simulink model "RealtimeModel"  (Simulink 7.0)
settings: Solver=FixedStepDiscrete  SolverMode=MultiTasking  StartTime=0.0  StopTime=RunningTime  FixedStep=sample  RelTol=1e-3
values from neighbouring files (symbols this model uses):
  Integrator = InitializeIntegrator(Integrator, Structure)    [RealtimeModel_Setup.m]
  SampleRate = Integrator.Timestep    [RealtimeModel_Setup.m]
  Structure = CalculateMatrices(Structure, Elements)    [RealtimeModel_Setup.m]
undefined symbols (not defined in the file or in its folder): Elements
libraries: simulink x2
(part 4 of 11)

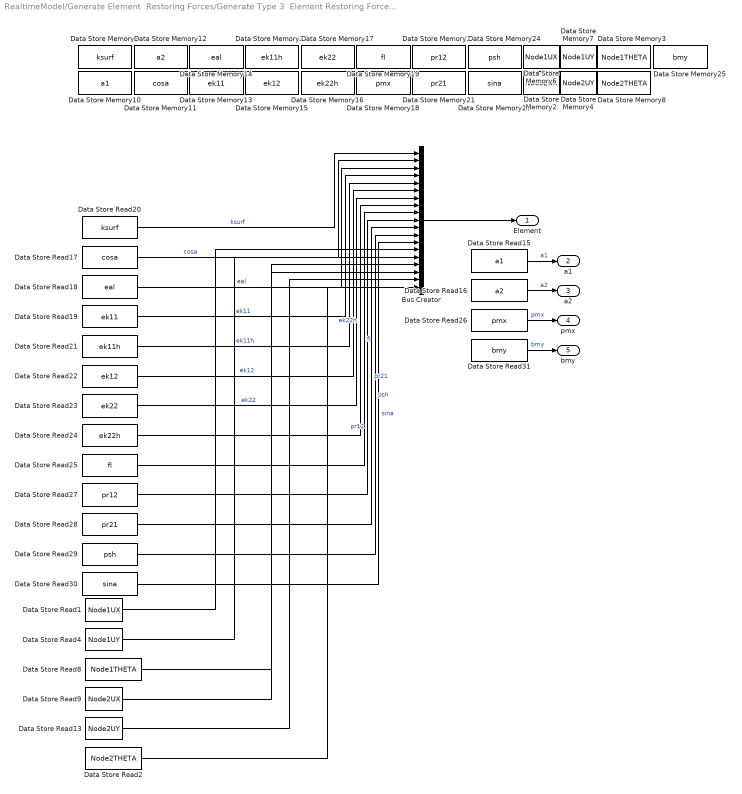
== system RealtimeModel/Generate Element  Restoring Forces/Generate Type 3  Element Restoring Force Element 19/Type 3 Element  ==
  Bus Creator : BusCreator  Inputs=19
  Data Store Memory10 : DataStoreMemory  DataStoreName=a1  InitialValue=Elements{id}.a1  OutDataType=sfix(16)  OutScaling=2^0
  Data Store Memory11 : DataStoreMemory  DataStoreName=cosa  InitialValue=Elements{id}.cosa  OutDataType=sfix(16)  OutScaling=2^0
  Data Store Memory12 : DataStoreMemory  DataStoreName=a2  InitialValue=Elements{id}.a2  OutDataType=sfix(16)  OutScaling=2^0
  Data Store Memory13 : DataStoreMemory  DataStoreName=ek11  InitialValue=Elements{id}.ek11  OutDataType=sfix(16)  OutScaling=2^0
  Data Store Memory14 : DataStoreMemory  DataStoreName=eal  InitialValue=Elements{id}.eal  OutDataType=sfix(16)  OutScaling=2^0
  Data Store Memory15 : DataStoreMemory  DataStoreName=ek12  InitialValue=Elements{id}.ek12  OutDataType=sfix(16)  OutScaling=2^0
  Data Store Memory16 : DataStoreMemory  DataStoreName=ek22h  InitialValue=Elements{id}.ek22h  OutDataType=sfix(16)  OutScaling=2^0
  Data Store Memory17 : DataStoreMemory  DataStoreName=ek22  InitialValue=Elements{id}.ek22  OutDataType=sfix(16)  OutScaling=2^0
  Data Store Memory18 : DataStoreMemory  DataStoreName=pmx  InitialValue=Elements{id}.pmx  OutDataType=sfix(16)  OutScaling=2^0
  Data Store Memory19 : DataStoreMemory  DataStoreName=fl  InitialValue=Elements{id}.fl  OutDataType=sfix(16)  OutScaling=2^0
  Data Store Memory2 : DataStoreMemory  DataStoreName=Node2UX  InitialValue=Elements{id}.Nodes(2).UX  OutDataType=sfix(16)  OutScaling=2^0
  Data Store Memory20 : DataStoreMemory  DataStoreName=ek11h  InitialValue=Elements{id}.ek11h  OutDataType=sfix(16)  OutScaling=2^0
  Data Store Memory21 : DataStoreMemory  DataStoreName=pr21  InitialValue=Elements{id}.pr21  OutDataType=sfix(16)  OutScaling=2^0
  Data Store Memory22 : DataStoreMemory  DataStoreName=pr12  InitialValue=Elements{id}.pr12  OutDataType=sfix(16)  OutScaling=2^0
  Data Store Memory23 : DataStoreMemory  DataStoreName=sina  InitialValue=Elements{id}.sina  OutDataType=sfix(16)  OutScaling=2^0
  Data Store Memory24 : DataStoreMemory  DataStoreName=psh  InitialValue=Elements{id}.psh  OutDataType=sfix(16)  OutScaling=2^0
  Data Store Memory25 : DataStoreMemory  DataStoreName=bmy  InitialValue=Elements{id}.bmy  OutDataType=sfix(16)  OutScaling=2^0
  Data Store Memory3 : DataStoreMemory  DataStoreName=Node1THETA  InitialValue=Elements{id}.Nodes(1).THETA  OutDataType=sfix(16)  OutScaling=2^0
  Data Store Memory4 : DataStoreMemory  DataStoreName=Node2UY  InitialValue=Elements{id}.Nodes(2).UY  OutDataType=sfix(16)  OutScaling=2^0
  Data Store Memory6 : DataStoreMemory  DataStoreName=Node1UX  InitialValue=Elements{id}.Nodes(1).UX  OutDataType=sfix(16)  OutScaling=2^0
  Data Store Memory7 : DataStoreMemory  DataStoreName=Node1UY  InitialValue=Elements{id}.Nodes(1).UY  OutDataType=sfix(16)  OutScaling=2^0
  Data Store Memory8 : DataStoreMemory  DataStoreName=Node2THETA  InitialValue=Elements{id}.Nodes(2).THETA  OutDataType=sfix(16)  OutScaling=2^0
  Data Store Memory9 : DataStoreMemory  DataStoreName=ksurf  InitialValue=Elements{id}.ksurf  OutDataType=sfix(16)  OutScaling=2^0
  Data Store Read1 : DataStoreRead  DataStoreName=Node1UX  SampleTime=-1
  Data Store Read13 : DataStoreRead  DataStoreName=Node2UY  SampleTime=-1
  Data Store Read15 : DataStoreRead  DataStoreName=a1  SampleTime=-1
  Data Store Read16 : DataStoreRead  DataStoreName=a2  SampleTime=-1
  Data Store Read17 : DataStoreRead  DataStoreName=cosa  SampleTime=-1
  Data Store Read18 : DataStoreRead  DataStoreName=eal  SampleTime=-1
  Data Store Read19 : DataStoreRead  DataStoreName=ek11  SampleTime=-1
  Data Store Read2 : DataStoreRead  DataStoreName=Node2THETA  SampleTime=-1
  Data Store Read20 : DataStoreRead  DataStoreName=ksurf  SampleTime=-1
  Data Store Read21 : DataStoreRead  DataStoreName=ek11h  SampleTime=-1
  Data Store Read22 : DataStoreRead  DataStoreName=ek12  SampleTime=-1
  Data Store Read23 : DataStoreRead  DataStoreName=ek22  SampleTime=-1
  Data Store Read24 : DataStoreRead  DataStoreName=ek22h  SampleTime=-1
  Data Store Read25 : DataStoreRead  DataStoreName=fl  SampleTime=-1
  Data Store Read26 : DataStoreRead  DataStoreName=pmx  SampleTime=-1
  Data Store Read27 : DataStoreRead  DataStoreName=pr12  SampleTime=-1
  Data Store Read28 : DataStoreRead  DataStoreName=pr21  SampleTime=-1
  Data Store Read29 : DataStoreRead  DataStoreName=psh  SampleTime=-1
  Data Store Read30 : DataStoreRead  DataStoreName=sina  SampleTime=-1
  Data Store Read31 : DataStoreRead  DataStoreName=bmy  SampleTime=-1
  Data Store Read4 : DataStoreRead  DataStoreName=Node1UY  SampleTime=-1
  Data Store Read8 : DataStoreRead  DataStoreName=Node1THETA  SampleTime=-1
  Data Store Read9 : DataStoreRead  DataStoreName=Node2UX  SampleTime=-1
  Element : Outport  OutDataType=sfix(16)  OutScaling=2^0
  a1 : Outport  Port=2  OutDataType=sfix(16)  OutScaling=2^0
  a2 : Outport  Port=3  OutDataType=sfix(16)  OutScaling=2^0
  pmx : Outport  Port=4  OutDataType=sfix(16)  OutScaling=2^0
  bmy : Outport  Port=5  OutDataType=sfix(16)  OutScaling=2^0
  wires:
  Data Store Read2/1 -> Bus Creator/19
  Data Store Read13/1 -> Bus Creator/18
  Data Store Read9/1 -> Bus Creator/17
  Data Store Read8/1 -> Bus Creator/16
  Data Store Read4/1 -> Bus Creator/15
  Data Store Read1/1 -> Bus Creator/14
  Bus Creator/1 -> Element/1
  Data Store Read20/1 -> Bus Creator/1  "ksurf"
  Data Store Read17/1 -> Bus Creator/2  "cosa"
  Data Store Read18/1 -> Bus Creator/3  "eal"
  Data Store Read19/1 -> Bus Creator/4  "ek11"
  Data Store Read21/1 -> Bus Creator/5  "ek11h"
  Data Store Read22/1 -> Bus Creator/6  "ek12"
  Data Store Read23/1 -> Bus Creator/7  "ek22"
  Data Store Read24/1 -> Bus Creator/8  "ek22h"
  Data Store Read25/1 -> Bus Creator/9  "fl"
  Data Store Read27/1 -> Bus Creator/10  "pr12"
  Data Store Read28/1 -> Bus Creator/11  "pr21"
  Data Store Read29/1 -> Bus Creator/12  "psh"
  Data Store Read30/1 -> Bus Creator/13  "sina"
  Data Store Read15/1 -> a1/1  "a1"
  Data Store Read16/1 -> a2/1  "a2"
  Data Store Read26/1 -> pmx/1  "pmx"
  Data Store Read31/1 -> bmy/1  "bmy"

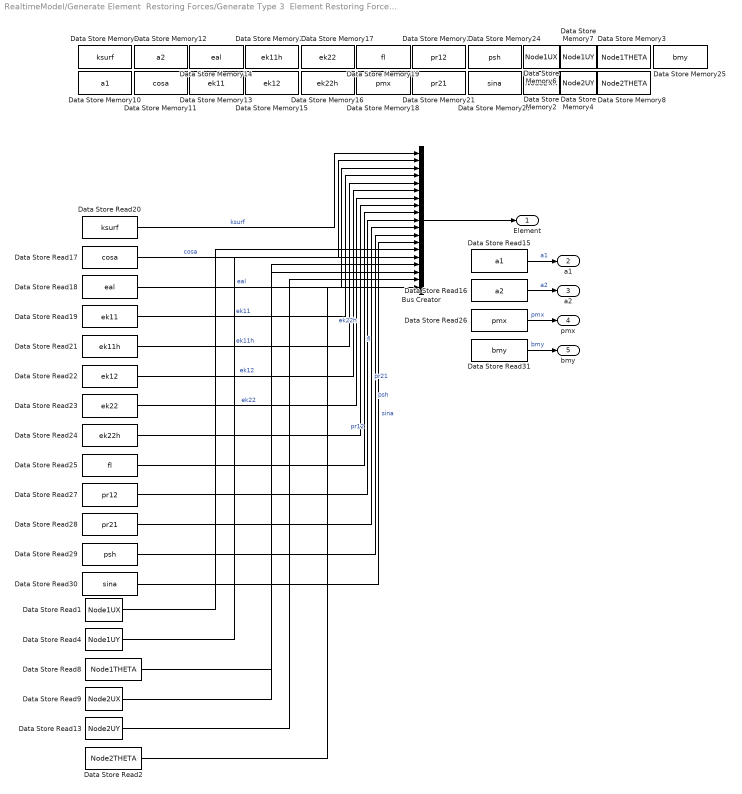
== system RealtimeModel/Generate Element  Restoring Forces/Generate Type 3  Element Restoring Force Element 2/Type 3 Element  ==
  Bus Creator : BusCreator  Inputs=19
  Data Store Memory10 : DataStoreMemory  DataStoreName=a1  InitialValue=Elements{id}.a1  OutDataType=sfix(16)  OutScaling=2^0
  Data Store Memory11 : DataStoreMemory  DataStoreName=cosa  InitialValue=Elements{id}.cosa  OutDataType=sfix(16)  OutScaling=2^0
  Data Store Memory12 : DataStoreMemory  DataStoreName=a2  InitialValue=Elements{id}.a2  OutDataType=sfix(16)  OutScaling=2^0
  Data Store Memory13 : DataStoreMemory  DataStoreName=ek11  InitialValue=Elements{id}.ek11  OutDataType=sfix(16)  OutScaling=2^0
  Data Store Memory14 : DataStoreMemory  DataStoreName=eal  InitialValue=Elements{id}.eal  OutDataType=sfix(16)  OutScaling=2^0
  Data Store Memory15 : DataStoreMemory  DataStoreName=ek12  InitialValue=Elements{id}.ek12  OutDataType=sfix(16)  OutScaling=2^0
  Data Store Memory16 : DataStoreMemory  DataStoreName=ek22h  InitialValue=Elements{id}.ek22h  OutDataType=sfix(16)  OutScaling=2^0
  Data Store Memory17 : DataStoreMemory  DataStoreName=ek22  InitialValue=Elements{id}.ek22  OutDataType=sfix(16)  OutScaling=2^0
  Data Store Memory18 : DataStoreMemory  DataStoreName=pmx  InitialValue=Elements{id}.pmx  OutDataType=sfix(16)  OutScaling=2^0
  Data Store Memory19 : DataStoreMemory  DataStoreName=fl  InitialValue=Elements{id}.fl  OutDataType=sfix(16)  OutScaling=2^0
  Data Store Memory2 : DataStoreMemory  DataStoreName=Node2UX  InitialValue=Elements{id}.Nodes(2).UX  OutDataType=sfix(16)  OutScaling=2^0
  Data Store Memory20 : DataStoreMemory  DataStoreName=ek11h  InitialValue=Elements{id}.ek11h  OutDataType=sfix(16)  OutScaling=2^0
  Data Store Memory21 : DataStoreMemory  DataStoreName=pr21  InitialValue=Elements{id}.pr21  OutDataType=sfix(16)  OutScaling=2^0
  Data Store Memory22 : DataStoreMemory  DataStoreName=pr12  InitialValue=Elements{id}.pr12  OutDataType=sfix(16)  OutScaling=2^0
  Data Store Memory23 : DataStoreMemory  DataStoreName=sina  InitialValue=Elements{id}.sina  OutDataType=sfix(16)  OutScaling=2^0
  Data Store Memory24 : DataStoreMemory  DataStoreName=psh  InitialValue=Elements{id}.psh  OutDataType=sfix(16)  OutScaling=2^0
  Data Store Memory25 : DataStoreMemory  DataStoreName=bmy  InitialValue=Elements{id}.bmy  OutDataType=sfix(16)  OutScaling=2^0
  Data Store Memory3 : DataStoreMemory  DataStoreName=Node1THETA  InitialValue=Elements{id}.Nodes(1).THETA  OutDataType=sfix(16)  OutScaling=2^0
  Data Store Memory4 : DataStoreMemory  DataStoreName=Node2UY  InitialValue=Elements{id}.Nodes(2).UY  OutDataType=sfix(16)  OutScaling=2^0
  Data Store Memory6 : DataStoreMemory  DataStoreName=Node1UX  InitialValue=Elements{id}.Nodes(1).UX  OutDataType=sfix(16)  OutScaling=2^0
  Data Store Memory7 : DataStoreMemory  DataStoreName=Node1UY  InitialValue=Elements{id}.Nodes(1).UY  OutDataType=sfix(16)  OutScaling=2^0
  Data Store Memory8 : DataStoreMemory  DataStoreName=Node2THETA  InitialValue=Elements{id}.Nodes(2).THETA  OutDataType=sfix(16)  OutScaling=2^0
  Data Store Memory9 : DataStoreMemory  DataStoreName=ksurf  InitialValue=Elements{id}.ksurf  OutDataType=sfix(16)  OutScaling=2^0
  Data Store Read1 : DataStoreRead  DataStoreName=Node1UX  SampleTime=-1
  Data Store Read13 : DataStoreRead  DataStoreName=Node2UY  SampleTime=-1
  Data Store Read15 : DataStoreRead  DataStoreName=a1  SampleTime=-1
  Data Store Read16 : DataStoreRead  DataStoreName=a2  SampleTime=-1
  Data Store Read17 : DataStoreRead  DataStoreName=cosa  SampleTime=-1
  Data Store Read18 : DataStoreRead  DataStoreName=eal  SampleTime=-1
  Data Store Read19 : DataStoreRead  DataStoreName=ek11  SampleTime=-1
  Data Store Read2 : DataStoreRead  DataStoreName=Node2THETA  SampleTime=-1
  Data Store Read20 : DataStoreRead  DataStoreName=ksurf  SampleTime=-1
  Data Store Read21 : DataStoreRead  DataStoreName=ek11h  SampleTime=-1
  Data Store Read22 : DataStoreRead  DataStoreName=ek12  SampleTime=-1
  Data Store Read23 : DataStoreRead  DataStoreName=ek22  SampleTime=-1
  Data Store Read24 : DataStoreRead  DataStoreName=ek22h  SampleTime=-1
  Data Store Read25 : DataStoreRead  DataStoreName=fl  SampleTime=-1
  Data Store Read26 : DataStoreRead  DataStoreName=pmx  SampleTime=-1
  Data Store Read27 : DataStoreRead  DataStoreName=pr12  SampleTime=-1
  Data Store Read28 : DataStoreRead  DataStoreName=pr21  SampleTime=-1
  Data Store Read29 : DataStoreRead  DataStoreName=psh  SampleTime=-1
  Data Store Read30 : DataStoreRead  DataStoreName=sina  SampleTime=-1
  Data Store Read31 : DataStoreRead  DataStoreName=bmy  SampleTime=-1
  Data Store Read4 : DataStoreRead  DataStoreName=Node1UY  SampleTime=-1
  Data Store Read8 : DataStoreRead  DataStoreName=Node1THETA  SampleTime=-1
  Data Store Read9 : DataStoreRead  DataStoreName=Node2UX  SampleTime=-1
  Element : Outport  OutDataType=sfix(16)  OutScaling=2^0
  a1 : Outport  Port=2  OutDataType=sfix(16)  OutScaling=2^0
  a2 : Outport  Port=3  OutDataType=sfix(16)  OutScaling=2^0
  pmx : Outport  Port=4  OutDataType=sfix(16)  OutScaling=2^0
  bmy : Outport  Port=5  OutDataType=sfix(16)  OutScaling=2^0
  wires:
  Data Store Read31/1 -> bmy/1  "bmy"
  Data Store Read26/1 -> pmx/1  "pmx"
  Data Store Read16/1 -> a2/1  "a2"
  Data Store Read15/1 -> a1/1  "a1"
  Data Store Read30/1 -> Bus Creator/13  "sina"
  Data Store Read29/1 -> Bus Creator/12  "psh"
  Data Store Read28/1 -> Bus Creator/11  "pr21"
  Data Store Read27/1 -> Bus Creator/10  "pr12"
  Data Store Read25/1 -> Bus Creator/9  "fl"
  Data Store Read24/1 -> Bus Creator/8  "ek22h"
  Data Store Read23/1 -> Bus Creator/7  "ek22"
  Data Store Read22/1 -> Bus Creator/6  "ek12"
  Data Store Read21/1 -> Bus Creator/5  "ek11h"
  Data Store Read19/1 -> Bus Creator/4  "ek11"
  Data Store Read18/1 -> Bus Creator/3  "eal"
  Data Store Read17/1 -> Bus Creator/2  "cosa"
  Data Store Read20/1 -> Bus Creator/1  "ksurf"
  Bus Creator/1 -> Element/1
  Data Store Read1/1 -> Bus Creator/14
  Data Store Read4/1 -> Bus Creator/15
  Data Store Read8/1 -> Bus Creator/16
  Data Store Read9/1 -> Bus Creator/17
  Data Store Read13/1 -> Bus Creator/18
  Data Store Read2/1 -> Bus Creator/19

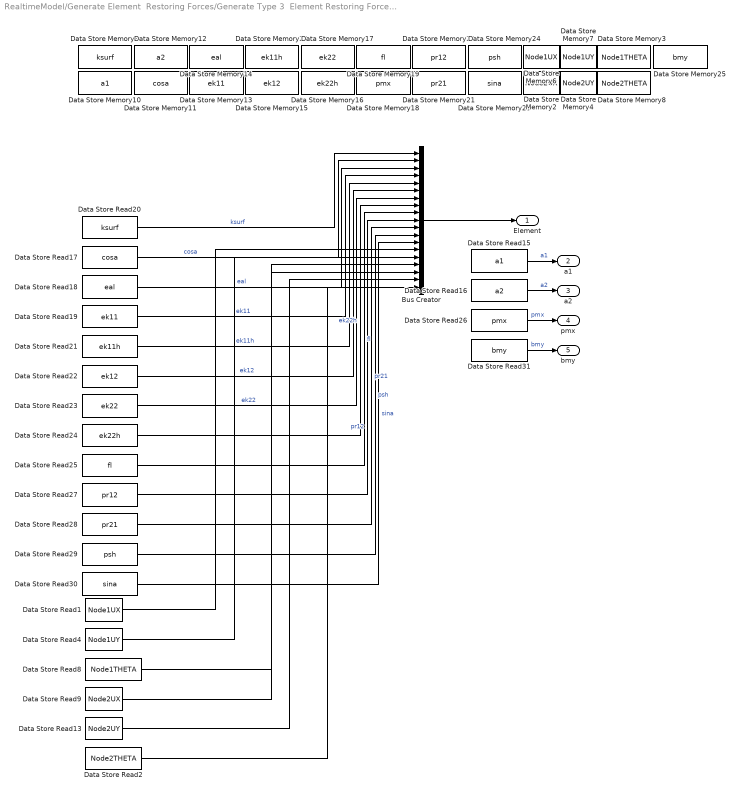
== system RealtimeModel/Generate Element  Restoring Forces/Generate Type 3  Element Restoring Force Element 21/Type 3 Element  ==
  Bus Creator : BusCreator  Inputs=19
  Data Store Memory10 : DataStoreMemory  DataStoreName=a1  InitialValue=Elements{id}.a1  OutDataType=sfix(16)  OutScaling=2^0
  Data Store Memory11 : DataStoreMemory  DataStoreName=cosa  InitialValue=Elements{id}.cosa  OutDataType=sfix(16)  OutScaling=2^0
  Data Store Memory12 : DataStoreMemory  DataStoreName=a2  InitialValue=Elements{id}.a2  OutDataType=sfix(16)  OutScaling=2^0
  Data Store Memory13 : DataStoreMemory  DataStoreName=ek11  InitialValue=Elements{id}.ek11  OutDataType=sfix(16)  OutScaling=2^0
  Data Store Memory14 : DataStoreMemory  DataStoreName=eal  InitialValue=Elements{id}.eal  OutDataType=sfix(16)  OutScaling=2^0
  Data Store Memory15 : DataStoreMemory  DataStoreName=ek12  InitialValue=Elements{id}.ek12  OutDataType=sfix(16)  OutScaling=2^0
  Data Store Memory16 : DataStoreMemory  DataStoreName=ek22h  InitialValue=Elements{id}.ek22h  OutDataType=sfix(16)  OutScaling=2^0
  Data Store Memory17 : DataStoreMemory  DataStoreName=ek22  InitialValue=Elements{id}.ek22  OutDataType=sfix(16)  OutScaling=2^0
  Data Store Memory18 : DataStoreMemory  DataStoreName=pmx  InitialValue=Elements{id}.pmx  OutDataType=sfix(16)  OutScaling=2^0
  Data Store Memory19 : DataStoreMemory  DataStoreName=fl  InitialValue=Elements{id}.fl  OutDataType=sfix(16)  OutScaling=2^0
  Data Store Memory2 : DataStoreMemory  DataStoreName=Node2UX  InitialValue=Elements{id}.Nodes(2).UX  OutDataType=sfix(16)  OutScaling=2^0
  Data Store Memory20 : DataStoreMemory  DataStoreName=ek11h  InitialValue=Elements{id}.ek11h  OutDataType=sfix(16)  OutScaling=2^0
  Data Store Memory21 : DataStoreMemory  DataStoreName=pr21  InitialValue=Elements{id}.pr21  OutDataType=sfix(16)  OutScaling=2^0
  Data Store Memory22 : DataStoreMemory  DataStoreName=pr12  InitialValue=Elements{id}.pr12  OutDataType=sfix(16)  OutScaling=2^0
  Data Store Memory23 : DataStoreMemory  DataStoreName=sina  InitialValue=Elements{id}.sina  OutDataType=sfix(16)  OutScaling=2^0
  Data Store Memory24 : DataStoreMemory  DataStoreName=psh  InitialValue=Elements{id}.psh  OutDataType=sfix(16)  OutScaling=2^0
  Data Store Memory25 : DataStoreMemory  DataStoreName=bmy  InitialValue=Elements{id}.bmy  OutDataType=sfix(16)  OutScaling=2^0
  Data Store Memory3 : DataStoreMemory  DataStoreName=Node1THETA  InitialValue=Elements{id}.Nodes(1).THETA  OutDataType=sfix(16)  OutScaling=2^0
  Data Store Memory4 : DataStoreMemory  DataStoreName=Node2UY  InitialValue=Elements{id}.Nodes(2).UY  OutDataType=sfix(16)  OutScaling=2^0
  Data Store Memory6 : DataStoreMemory  DataStoreName=Node1UX  InitialValue=Elements{id}.Nodes(1).UX  OutDataType=sfix(16)  OutScaling=2^0
  Data Store Memory7 : DataStoreMemory  DataStoreName=Node1UY  InitialValue=Elements{id}.Nodes(1).UY  OutDataType=sfix(16)  OutScaling=2^0
  Data Store Memory8 : DataStoreMemory  DataStoreName=Node2THETA  InitialValue=Elements{id}.Nodes(2).THETA  OutDataType=sfix(16)  OutScaling=2^0
  Data Store Memory9 : DataStoreMemory  DataStoreName=ksurf  InitialValue=Elements{id}.ksurf  OutDataType=sfix(16)  OutScaling=2^0
  Data Store Read1 : DataStoreRead  DataStoreName=Node1UX  SampleTime=-1
  Data Store Read13 : DataStoreRead  DataStoreName=Node2UY  SampleTime=-1
  Data Store Read15 : DataStoreRead  DataStoreName=a1  SampleTime=-1
  Data Store Read16 : DataStoreRead  DataStoreName=a2  SampleTime=-1
  Data Store Read17 : DataStoreRead  DataStoreName=cosa  SampleTime=-1
  Data Store Read18 : DataStoreRead  DataStoreName=eal  SampleTime=-1
  Data Store Read19 : DataStoreRead  DataStoreName=ek11  SampleTime=-1
  Data Store Read2 : DataStoreRead  DataStoreName=Node2THETA  SampleTime=-1
  Data Store Read20 : DataStoreRead  DataStoreName=ksurf  SampleTime=-1
  Data Store Read21 : DataStoreRead  DataStoreName=ek11h  SampleTime=-1
  Data Store Read22 : DataStoreRead  DataStoreName=ek12  SampleTime=-1
  Data Store Read23 : DataStoreRead  DataStoreName=ek22  SampleTime=-1
  Data Store Read24 : DataStoreRead  DataStoreName=ek22h  SampleTime=-1
  Data Store Read25 : DataStoreRead  DataStoreName=fl  SampleTime=-1
  Data Store Read26 : DataStoreRead  DataStoreName=pmx  SampleTime=-1
  Data Store Read27 : DataStoreRead  DataStoreName=pr12  SampleTime=-1
  Data Store Read28 : DataStoreRead  DataStoreName=pr21  SampleTime=-1
  Data Store Read29 : DataStoreRead  DataStoreName=psh  SampleTime=-1
  Data Store Read30 : DataStoreRead  DataStoreName=sina  SampleTime=-1
  Data Store Read31 : DataStoreRead  DataStoreName=bmy  SampleTime=-1
  Data Store Read4 : DataStoreRead  DataStoreName=Node1UY  SampleTime=-1
  Data Store Read8 : DataStoreRead  DataStoreName=Node1THETA  SampleTime=-1
  Data Store Read9 : DataStoreRead  DataStoreName=Node2UX  SampleTime=-1
  Element : Outport  OutDataType=sfix(16)  OutScaling=2^0
  a1 : Outport  Port=2  OutDataType=sfix(16)  OutScaling=2^0
  a2 : Outport  Port=3  OutDataType=sfix(16)  OutScaling=2^0
  pmx : Outport  Port=4  OutDataType=sfix(16)  OutScaling=2^0
  bmy : Outport  Port=5  OutDataType=sfix(16)  OutScaling=2^0
  wires:
  Data Store Read2/1 -> Bus Creator/19
  Data Store Read13/1 -> Bus Creator/18
  Data Store Read9/1 -> Bus Creator/17
  Data Store Read8/1 -> Bus Creator/16
  Data Store Read4/1 -> Bus Creator/15
  Data Store Read1/1 -> Bus Creator/14
  Bus Creator/1 -> Element/1
  Data Store Read20/1 -> Bus Creator/1  "ksurf"
  Data Store Read17/1 -> Bus Creator/2  "cosa"
  Data Store Read18/1 -> Bus Creator/3  "eal"
  Data Store Read19/1 -> Bus Creator/4  "ek11"
  Data Store Read21/1 -> Bus Creator/5  "ek11h"
  Data Store Read22/1 -> Bus Creator/6  "ek12"
  Data Store Read23/1 -> Bus Creator/7  "ek22"
  Data Store Read24/1 -> Bus Creator/8  "ek22h"
  Data Store Read25/1 -> Bus Creator/9  "fl"
  Data Store Read27/1 -> Bus Creator/10  "pr12"
  Data Store Read28/1 -> Bus Creator/11  "pr21"
  Data Store Read29/1 -> Bus Creator/12  "psh"
  Data Store Read30/1 -> Bus Creator/13  "sina"
  Data Store Read15/1 -> a1/1  "a1"
  Data Store Read16/1 -> a2/1  "a2"
  Data Store Read26/1 -> pmx/1  "pmx"
  Data Store Read31/1 -> bmy/1  "bmy"

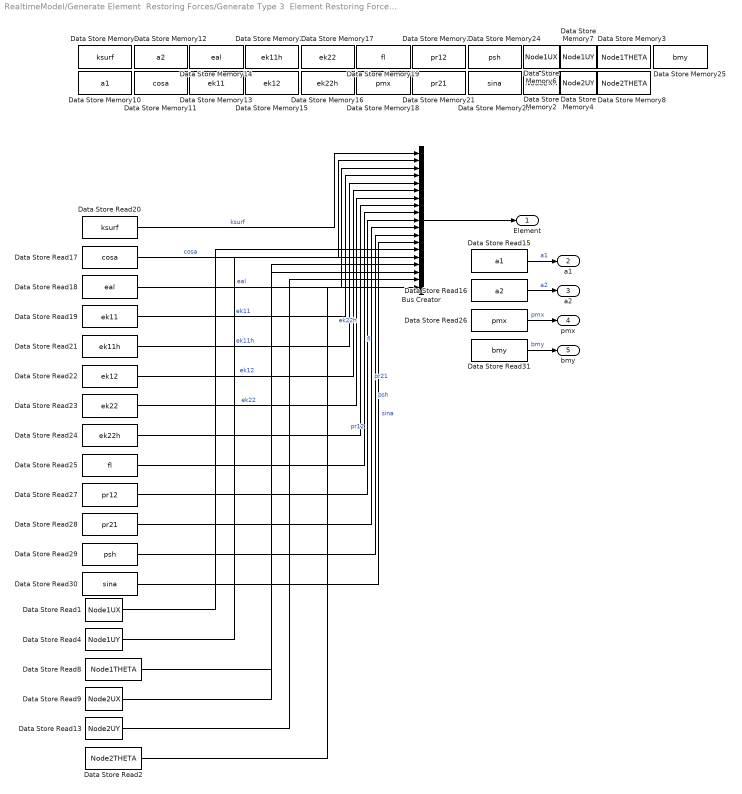
== system RealtimeModel/Generate Element  Restoring Forces/Generate Type 3  Element Restoring Force Element 22/Type 3 Element  ==
  Bus Creator : BusCreator  Inputs=19
  Data Store Memory10 : DataStoreMemory  DataStoreName=a1  InitialValue=Elements{id}.a1  OutDataType=sfix(16)  OutScaling=2^0
  Data Store Memory11 : DataStoreMemory  DataStoreName=cosa  InitialValue=Elements{id}.cosa  OutDataType=sfix(16)  OutScaling=2^0
  Data Store Memory12 : DataStoreMemory  DataStoreName=a2  InitialValue=Elements{id}.a2  OutDataType=sfix(16)  OutScaling=2^0
  Data Store Memory13 : DataStoreMemory  DataStoreName=ek11  InitialValue=Elements{id}.ek11  OutDataType=sfix(16)  OutScaling=2^0
  Data Store Memory14 : DataStoreMemory  DataStoreName=eal  InitialValue=Elements{id}.eal  OutDataType=sfix(16)  OutScaling=2^0
  Data Store Memory15 : DataStoreMemory  DataStoreName=ek12  InitialValue=Elements{id}.ek12  OutDataType=sfix(16)  OutScaling=2^0
  Data Store Memory16 : DataStoreMemory  DataStoreName=ek22h  InitialValue=Elements{id}.ek22h  OutDataType=sfix(16)  OutScaling=2^0
  Data Store Memory17 : DataStoreMemory  DataStoreName=ek22  InitialValue=Elements{id}.ek22  OutDataType=sfix(16)  OutScaling=2^0
  Data Store Memory18 : DataStoreMemory  DataStoreName=pmx  InitialValue=Elements{id}.pmx  OutDataType=sfix(16)  OutScaling=2^0
  Data Store Memory19 : DataStoreMemory  DataStoreName=fl  InitialValue=Elements{id}.fl  OutDataType=sfix(16)  OutScaling=2^0
  Data Store Memory2 : DataStoreMemory  DataStoreName=Node2UX  InitialValue=Elements{id}.Nodes(2).UX  OutDataType=sfix(16)  OutScaling=2^0
  Data Store Memory20 : DataStoreMemory  DataStoreName=ek11h  InitialValue=Elements{id}.ek11h  OutDataType=sfix(16)  OutScaling=2^0
  Data Store Memory21 : DataStoreMemory  DataStoreName=pr21  InitialValue=Elements{id}.pr21  OutDataType=sfix(16)  OutScaling=2^0
  Data Store Memory22 : DataStoreMemory  DataStoreName=pr12  InitialValue=Elements{id}.pr12  OutDataType=sfix(16)  OutScaling=2^0
  Data Store Memory23 : DataStoreMemory  DataStoreName=sina  InitialValue=Elements{id}.sina  OutDataType=sfix(16)  OutScaling=2^0
  Data Store Memory24 : DataStoreMemory  DataStoreName=psh  InitialValue=Elements{id}.psh  OutDataType=sfix(16)  OutScaling=2^0
  Data Store Memory25 : DataStoreMemory  DataStoreName=bmy  InitialValue=Elements{id}.bmy  OutDataType=sfix(16)  OutScaling=2^0
  Data Store Memory3 : DataStoreMemory  DataStoreName=Node1THETA  InitialValue=Elements{id}.Nodes(1).THETA  OutDataType=sfix(16)  OutScaling=2^0
  Data Store Memory4 : DataStoreMemory  DataStoreName=Node2UY  InitialValue=Elements{id}.Nodes(2).UY  OutDataType=sfix(16)  OutScaling=2^0
  Data Store Memory6 : DataStoreMemory  DataStoreName=Node1UX  InitialValue=Elements{id}.Nodes(1).UX  OutDataType=sfix(16)  OutScaling=2^0
  Data Store Memory7 : DataStoreMemory  DataStoreName=Node1UY  InitialValue=Elements{id}.Nodes(1).UY  OutDataType=sfix(16)  OutScaling=2^0
  Data Store Memory8 : DataStoreMemory  DataStoreName=Node2THETA  InitialValue=Elements{id}.Nodes(2).THETA  OutDataType=sfix(16)  OutScaling=2^0
  Data Store Memory9 : DataStoreMemory  DataStoreName=ksurf  InitialValue=Elements{id}.ksurf  OutDataType=sfix(16)  OutScaling=2^0
  Data Store Read1 : DataStoreRead  DataStoreName=Node1UX  SampleTime=-1
  Data Store Read13 : DataStoreRead  DataStoreName=Node2UY  SampleTime=-1
  Data Store Read15 : DataStoreRead  DataStoreName=a1  SampleTime=-1
  Data Store Read16 : DataStoreRead  DataStoreName=a2  SampleTime=-1
  Data Store Read17 : DataStoreRead  DataStoreName=cosa  SampleTime=-1
  Data Store Read18 : DataStoreRead  DataStoreName=eal  SampleTime=-1
  Data Store Read19 : DataStoreRead  DataStoreName=ek11  SampleTime=-1
  Data Store Read2 : DataStoreRead  DataStoreName=Node2THETA  SampleTime=-1
  Data Store Read20 : DataStoreRead  DataStoreName=ksurf  SampleTime=-1
  Data Store Read21 : DataStoreRead  DataStoreName=ek11h  SampleTime=-1
  Data Store Read22 : DataStoreRead  DataStoreName=ek12  SampleTime=-1
  Data Store Read23 : DataStoreRead  DataStoreName=ek22  SampleTime=-1
  Data Store Read24 : DataStoreRead  DataStoreName=ek22h  SampleTime=-1
  Data Store Read25 : DataStoreRead  DataStoreName=fl  SampleTime=-1
  Data Store Read26 : DataStoreRead  DataStoreName=pmx  SampleTime=-1
  Data Store Read27 : DataStoreRead  DataStoreName=pr12  SampleTime=-1
  Data Store Read28 : DataStoreRead  DataStoreName=pr21  SampleTime=-1
  Data Store Read29 : DataStoreRead  DataStoreName=psh  SampleTime=-1
  Data Store Read30 : DataStoreRead  DataStoreName=sina  SampleTime=-1
  Data Store Read31 : DataStoreRead  DataStoreName=bmy  SampleTime=-1
  Data Store Read4 : DataStoreRead  DataStoreName=Node1UY  SampleTime=-1
  Data Store Read8 : DataStoreRead  DataStoreName=Node1THETA  SampleTime=-1
  Data Store Read9 : DataStoreRead  DataStoreName=Node2UX  SampleTime=-1
  Element : Outport  OutDataType=sfix(16)  OutScaling=2^0
  a1 : Outport  Port=2  OutDataType=sfix(16)  OutScaling=2^0
  a2 : Outport  Port=3  OutDataType=sfix(16)  OutScaling=2^0
  pmx : Outport  Port=4  OutDataType=sfix(16)  OutScaling=2^0
  bmy : Outport  Port=5  OutDataType=sfix(16)  OutScaling=2^0
  wires:
  Data Store Read31/1 -> bmy/1  "bmy"
  Data Store Read26/1 -> pmx/1  "pmx"
  Data Store Read16/1 -> a2/1  "a2"
  Data Store Read15/1 -> a1/1  "a1"
  Data Store Read30/1 -> Bus Creator/13  "sina"
  Data Store Read29/1 -> Bus Creator/12  "psh"
  Data Store Read28/1 -> Bus Creator/11  "pr21"
  Data Store Read27/1 -> Bus Creator/10  "pr12"
  Data Store Read25/1 -> Bus Creator/9  "fl"
  Data Store Read24/1 -> Bus Creator/8  "ek22h"
  Data Store Read23/1 -> Bus Creator/7  "ek22"
  Data Store Read22/1 -> Bus Creator/6  "ek12"
  Data Store Read21/1 -> Bus Creator/5  "ek11h"
  Data Store Read19/1 -> Bus Creator/4  "ek11"
  Data Store Read18/1 -> Bus Creator/3  "eal"
  Data Store Read17/1 -> Bus Creator/2  "cosa"
  Data Store Read20/1 -> Bus Creator/1  "ksurf"
  Bus Creator/1 -> Element/1
  Data Store Read1/1 -> Bus Creator/14
  Data Store Read4/1 -> Bus Creator/15
  Data Store Read8/1 -> Bus Creator/16
  Data Store Read9/1 -> Bus Creator/17
  Data Store Read13/1 -> Bus Creator/18
  Data Store Read2/1 -> Bus Creator/19

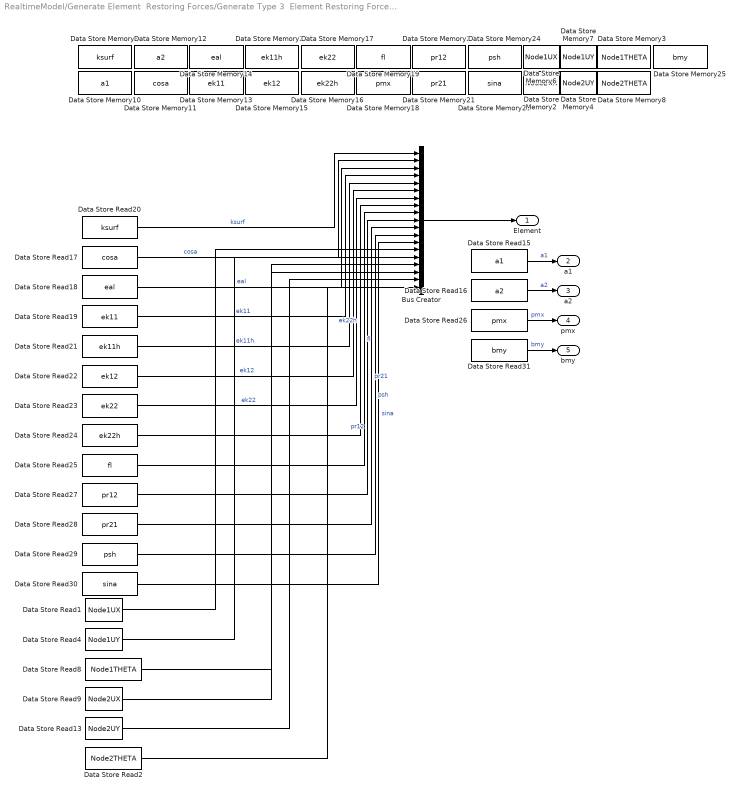
== system RealtimeModel/Generate Element  Restoring Forces/Generate Type 3  Element Restoring Force Element 24/Type 3 Element  ==
  Bus Creator : BusCreator  Inputs=19
  Data Store Memory10 : DataStoreMemory  DataStoreName=a1  InitialValue=Elements{id}.a1  OutDataType=sfix(16)  OutScaling=2^0
  Data Store Memory11 : DataStoreMemory  DataStoreName=cosa  InitialValue=Elements{id}.cosa  OutDataType=sfix(16)  OutScaling=2^0
  Data Store Memory12 : DataStoreMemory  DataStoreName=a2  InitialValue=Elements{id}.a2  OutDataType=sfix(16)  OutScaling=2^0
  Data Store Memory13 : DataStoreMemory  DataStoreName=ek11  InitialValue=Elements{id}.ek11  OutDataType=sfix(16)  OutScaling=2^0
  Data Store Memory14 : DataStoreMemory  DataStoreName=eal  InitialValue=Elements{id}.eal  OutDataType=sfix(16)  OutScaling=2^0
  Data Store Memory15 : DataStoreMemory  DataStoreName=ek12  InitialValue=Elements{id}.ek12  OutDataType=sfix(16)  OutScaling=2^0
  Data Store Memory16 : DataStoreMemory  DataStoreName=ek22h  InitialValue=Elements{id}.ek22h  OutDataType=sfix(16)  OutScaling=2^0
  Data Store Memory17 : DataStoreMemory  DataStoreName=ek22  InitialValue=Elements{id}.ek22  OutDataType=sfix(16)  OutScaling=2^0
  Data Store Memory18 : DataStoreMemory  DataStoreName=pmx  InitialValue=Elements{id}.pmx  OutDataType=sfix(16)  OutScaling=2^0
  Data Store Memory19 : DataStoreMemory  DataStoreName=fl  InitialValue=Elements{id}.fl  OutDataType=sfix(16)  OutScaling=2^0
  Data Store Memory2 : DataStoreMemory  DataStoreName=Node2UX  InitialValue=Elements{id}.Nodes(2).UX  OutDataType=sfix(16)  OutScaling=2^0
  Data Store Memory20 : DataStoreMemory  DataStoreName=ek11h  InitialValue=Elements{id}.ek11h  OutDataType=sfix(16)  OutScaling=2^0
  Data Store Memory21 : DataStoreMemory  DataStoreName=pr21  InitialValue=Elements{id}.pr21  OutDataType=sfix(16)  OutScaling=2^0
  Data Store Memory22 : DataStoreMemory  DataStoreName=pr12  InitialValue=Elements{id}.pr12  OutDataType=sfix(16)  OutScaling=2^0
  Data Store Memory23 : DataStoreMemory  DataStoreName=sina  InitialValue=Elements{id}.sina  OutDataType=sfix(16)  OutScaling=2^0
  Data Store Memory24 : DataStoreMemory  DataStoreName=psh  InitialValue=Elements{id}.psh  OutDataType=sfix(16)  OutScaling=2^0
  Data Store Memory25 : DataStoreMemory  DataStoreName=bmy  InitialValue=Elements{id}.bmy  OutDataType=sfix(16)  OutScaling=2^0
  Data Store Memory3 : DataStoreMemory  DataStoreName=Node1THETA  InitialValue=Elements{id}.Nodes(1).THETA  OutDataType=sfix(16)  OutScaling=2^0
  Data Store Memory4 : DataStoreMemory  DataStoreName=Node2UY  InitialValue=Elements{id}.Nodes(2).UY  OutDataType=sfix(16)  OutScaling=2^0
  Data Store Memory6 : DataStoreMemory  DataStoreName=Node1UX  InitialValue=Elements{id}.Nodes(1).UX  OutDataType=sfix(16)  OutScaling=2^0
  Data Store Memory7 : DataStoreMemory  DataStoreName=Node1UY  InitialValue=Elements{id}.Nodes(1).UY  OutDataType=sfix(16)  OutScaling=2^0
  Data Store Memory8 : DataStoreMemory  DataStoreName=Node2THETA  InitialValue=Elements{id}.Nodes(2).THETA  OutDataType=sfix(16)  OutScaling=2^0
  Data Store Memory9 : DataStoreMemory  DataStoreName=ksurf  InitialValue=Elements{id}.ksurf  OutDataType=sfix(16)  OutScaling=2^0
  Data Store Read1 : DataStoreRead  DataStoreName=Node1UX  SampleTime=-1
  Data Store Read13 : DataStoreRead  DataStoreName=Node2UY  SampleTime=-1
  Data Store Read15 : DataStoreRead  DataStoreName=a1  SampleTime=-1
  Data Store Read16 : DataStoreRead  DataStoreName=a2  SampleTime=-1
  Data Store Read17 : DataStoreRead  DataStoreName=cosa  SampleTime=-1
  Data Store Read18 : DataStoreRead  DataStoreName=eal  SampleTime=-1
  Data Store Read19 : DataStoreRead  DataStoreName=ek11  SampleTime=-1
  Data Store Read2 : DataStoreRead  DataStoreName=Node2THETA  SampleTime=-1
  Data Store Read20 : DataStoreRead  DataStoreName=ksurf  SampleTime=-1
  Data Store Read21 : DataStoreRead  DataStoreName=ek11h  SampleTime=-1
  Data Store Read22 : DataStoreRead  DataStoreName=ek12  SampleTime=-1
  Data Store Read23 : DataStoreRead  DataStoreName=ek22  SampleTime=-1
  Data Store Read24 : DataStoreRead  DataStoreName=ek22h  SampleTime=-1
  Data Store Read25 : DataStoreRead  DataStoreName=fl  SampleTime=-1
  Data Store Read26 : DataStoreRead  DataStoreName=pmx  SampleTime=-1
  Data Store Read27 : DataStoreRead  DataStoreName=pr12  SampleTime=-1
  Data Store Read28 : DataStoreRead  DataStoreName=pr21  SampleTime=-1
  Data Store Read29 : DataStoreRead  DataStoreName=psh  SampleTime=-1
  Data Store Read30 : DataStoreRead  DataStoreName=sina  SampleTime=-1
  Data Store Read31 : DataStoreRead  DataStoreName=bmy  SampleTime=-1
  Data Store Read4 : DataStoreRead  DataStoreName=Node1UY  SampleTime=-1
  Data Store Read8 : DataStoreRead  DataStoreName=Node1THETA  SampleTime=-1
  Data Store Read9 : DataStoreRead  DataStoreName=Node2UX  SampleTime=-1
  Element : Outport  OutDataType=sfix(16)  OutScaling=2^0
  a1 : Outport  Port=2  OutDataType=sfix(16)  OutScaling=2^0
  a2 : Outport  Port=3  OutDataType=sfix(16)  OutScaling=2^0
  pmx : Outport  Port=4  OutDataType=sfix(16)  OutScaling=2^0
  bmy : Outport  Port=5  OutDataType=sfix(16)  OutScaling=2^0
  wires:
  Data Store Read2/1 -> Bus Creator/19
  Data Store Read13/1 -> Bus Creator/18
  Data Store Read9/1 -> Bus Creator/17
  Data Store Read8/1 -> Bus Creator/16
  Data Store Read4/1 -> Bus Creator/15
  Data Store Read1/1 -> Bus Creator/14
  Bus Creator/1 -> Element/1
  Data Store Read20/1 -> Bus Creator/1  "ksurf"
  Data Store Read17/1 -> Bus Creator/2  "cosa"
  Data Store Read18/1 -> Bus Creator/3  "eal"
  Data Store Read19/1 -> Bus Creator/4  "ek11"
  Data Store Read21/1 -> Bus Creator/5  "ek11h"
  Data Store Read22/1 -> Bus Creator/6  "ek12"
  Data Store Read23/1 -> Bus Creator/7  "ek22"
  Data Store Read24/1 -> Bus Creator/8  "ek22h"
  Data Store Read25/1 -> Bus Creator/9  "fl"
  Data Store Read27/1 -> Bus Creator/10  "pr12"
  Data Store Read28/1 -> Bus Creator/11  "pr21"
  Data Store Read29/1 -> Bus Creator/12  "psh"
  Data Store Read30/1 -> Bus Creator/13  "sina"
  Data Store Read15/1 -> a1/1  "a1"
  Data Store Read16/1 -> a2/1  "a2"
  Data Store Read26/1 -> pmx/1  "pmx"
  Data Store Read31/1 -> bmy/1  "bmy"

== system RealtimeModel/Generate Element  Restoring Forces/Generate Type 3  Element Restoring Force Element 25/Type 3 Element  ==
  Bus Creator : BusCreator  Inputs=19
  Data Store Memory10 : DataStoreMemory  DataStoreName=a1  InitialValue=Elements{id}.a1  OutDataType=sfix(16)  OutScaling=2^0
  Data Store Memory11 : DataStoreMemory  DataStoreName=cosa  InitialValue=Elements{id}.cosa  OutDataType=sfix(16)  OutScaling=2^0
  Data Store Memory12 : DataStoreMemory  DataStoreName=a2  InitialValue=Elements{id}.a2  OutDataType=sfix(16)  OutScaling=2^0
  Data Store Memory13 : DataStoreMemory  DataStoreName=ek11  InitialValue=Elements{id}.ek11  OutDataType=sfix(16)  OutScaling=2^0
  Data Store Memory14 : DataStoreMemory  DataStoreName=eal  InitialValue=Elements{id}.eal  OutDataType=sfix(16)  OutScaling=2^0
  Data Store Memory15 : DataStoreMemory  DataStoreName=ek12  InitialValue=Elements{id}.ek12  OutDataType=sfix(16)  OutScaling=2^0
  Data Store Memory16 : DataStoreMemory  DataStoreName=ek22h  InitialValue=Elements{id}.ek22h  OutDataType=sfix(16)  OutScaling=2^0
  Data Store Memory17 : DataStoreMemory  DataStoreName=ek22  InitialValue=Elements{id}.ek22  OutDataType=sfix(16)  OutScaling=2^0
  Data Store Memory18 : DataStoreMemory  DataStoreName=pmx  InitialValue=Elements{id}.pmx  OutDataType=sfix(16)  OutScaling=2^0
  Data Store Memory19 : DataStoreMemory  DataStoreName=fl  InitialValue=Elements{id}.fl  OutDataType=sfix(16)  OutScaling=2^0
  Data Store Memory2 : DataStoreMemory  DataStoreName=Node2UX  InitialValue=Elements{id}.Nodes(2).UX  OutDataType=sfix(16)  OutScaling=2^0
  Data Store Memory20 : DataStoreMemory  DataStoreName=ek11h  InitialValue=Elements{id}.ek11h  OutDataType=sfix(16)  OutScaling=2^0
  Data Store Memory21 : DataStoreMemory  DataStoreName=pr21  InitialValue=Elements{id}.pr21  OutDataType=sfix(16)  OutScaling=2^0
  Data Store Memory22 : DataStoreMemory  DataStoreName=pr12  InitialValue=Elements{id}.pr12  OutDataType=sfix(16)  OutScaling=2^0
  Data Store Memory23 : DataStoreMemory  DataStoreName=sina  InitialValue=Elements{id}.sina  OutDataType=sfix(16)  OutScaling=2^0
  Data Store Memory24 : DataStoreMemory  DataStoreName=psh  InitialValue=Elements{id}.psh  OutDataType=sfix(16)  OutScaling=2^0
  Data Store Memory25 : DataStoreMemory  DataStoreName=bmy  InitialValue=Elements{id}.bmy  OutDataType=sfix(16)  OutScaling=2^0
  Data Store Memory3 : DataStoreMemory  DataStoreName=Node1THETA  InitialValue=Elements{id}.Nodes(1).THETA  OutDataType=sfix(16)  OutScaling=2^0
  Data Store Memory4 : DataStoreMemory  DataStoreName=Node2UY  InitialValue=Elements{id}.Nodes(2).UY  OutDataType=sfix(16)  OutScaling=2^0
  Data Store Memory6 : DataStoreMemory  DataStoreName=Node1UX  InitialValue=Elements{id}.Nodes(1).UX  OutDataType=sfix(16)  OutScaling=2^0
  Data Store Memory7 : DataStoreMemory  DataStoreName=Node1UY  InitialValue=Elements{id}.Nodes(1).UY  OutDataType=sfix(16)  OutScaling=2^0
  Data Store Memory8 : DataStoreMemory  DataStoreName=Node2THETA  InitialValue=Elements{id}.Nodes(2).THETA  OutDataType=sfix(16)  OutScaling=2^0
  Data Store Memory9 : DataStoreMemory  DataStoreName=ksurf  InitialValue=Elements{id}.ksurf  OutDataType=sfix(16)  OutScaling=2^0
  Data Store Read1 : DataStoreRead  DataStoreName=Node1UX  SampleTime=-1
  Data Store Read13 : DataStoreRead  DataStoreName=Node2UY  SampleTime=-1
  Data Store Read15 : DataStoreRead  DataStoreName=a1  SampleTime=-1
  Data Store Read16 : DataStoreRead  DataStoreName=a2  SampleTime=-1
  Data Store Read17 : DataStoreRead  DataStoreName=cosa  SampleTime=-1
  Data Store Read18 : DataStoreRead  DataStoreName=eal  SampleTime=-1
  Data Store Read19 : DataStoreRead  DataStoreName=ek11  SampleTime=-1
  Data Store Read2 : DataStoreRead  DataStoreName=Node2THETA  SampleTime=-1
  Data Store Read20 : DataStoreRead  DataStoreName=ksurf  SampleTime=-1
  Data Store Read21 : DataStoreRead  DataStoreName=ek11h  SampleTime=-1
  Data Store Read22 : DataStoreRead  DataStoreName=ek12  SampleTime=-1
  Data Store Read23 : DataStoreRead  DataStoreName=ek22  SampleTime=-1
  Data Store Read24 : DataStoreRead  DataStoreName=ek22h  SampleTime=-1
  Data Store Read25 : DataStoreRead  DataStoreName=fl  SampleTime=-1
  Data Store Read26 : DataStoreRead  DataStoreName=pmx  SampleTime=-1
  Data Store Read27 : DataStoreRead  DataStoreName=pr12  SampleTime=-1
  Data Store Read28 : DataStoreRead  DataStoreName=pr21  SampleTime=-1
  Data Store Read29 : DataStoreRead  DataStoreName=psh  SampleTime=-1
  Data Store Read30 : DataStoreRead  DataStoreName=sina  SampleTime=-1
  Data Store Read31 : DataStoreRead  DataStoreName=bmy  SampleTime=-1
  Data Store Read4 : DataStoreRead  DataStoreName=Node1UY  SampleTime=-1
  Data Store Read8 : DataStoreRead  DataStoreName=Node1THETA  SampleTime=-1
  Data Store Read9 : DataStoreRead  DataStoreName=Node2UX  SampleTime=-1
  Element : Outport  OutDataType=sfix(16)  OutScaling=2^0
  a1 : Outport  Port=2  OutDataType=sfix(16)  OutScaling=2^0
  a2 : Outport  Port=3  OutDataType=sfix(16)  OutScaling=2^0
  pmx : Outport  Port=4  OutDataType=sfix(16)  OutScaling=2^0
  bmy : Outport  Port=5  OutDataType=sfix(16)  OutScaling=2^0
  wires:
  Data Store Read2/1 -> Bus Creator/19
  Data Store Read13/1 -> Bus Creator/18
  Data Store Read9/1 -> Bus Creator/17
  Data Store Read8/1 -> Bus Creator/16
  Data Store Read4/1 -> Bus Creator/15
  Data Store Read1/1 -> Bus Creator/14
  Bus Creator/1 -> Element/1
  Data Store Read20/1 -> Bus Creator/1  "ksurf"
  Data Store Read17/1 -> Bus Creator/2  "cosa"
  Data Store Read18/1 -> Bus Creator/3  "eal"
  Data Store Read19/1 -> Bus Creator/4  "ek11"
  Data Store Read21/1 -> Bus Creator/5  "ek11h"
  Data Store Read22/1 -> Bus Creator/6  "ek12"
  Data Store Read23/1 -> Bus Creator/7  "ek22"
  Data Store Read24/1 -> Bus Creator/8  "ek22h"
  Data Store Read25/1 -> Bus Creator/9  "fl"
  Data Store Read27/1 -> Bus Creator/10  "pr12"
  Data Store Read28/1 -> Bus Creator/11  "pr21"
  Data Store Read29/1 -> Bus Creator/12  "psh"
  Data Store Read30/1 -> Bus Creator/13  "sina"
  Data Store Read15/1 -> a1/1  "a1"
  Data Store Read16/1 -> a2/1  "a2"
  Data Store Read26/1 -> pmx/1  "pmx"
  Data Store Read31/1 -> bmy/1  "bmy"

== system RealtimeModel/Generate Element  Restoring Forces/Generate Type 3  Element Restoring Force Element 26/Type 3 Element  ==
  Bus Creator : BusCreator  Inputs=19
  Data Store Memory10 : DataStoreMemory  DataStoreName=a1  InitialValue=Elements{id}.a1  OutDataType=sfix(16)  OutScaling=2^0
  Data Store Memory11 : DataStoreMemory  DataStoreName=cosa  InitialValue=Elements{id}.cosa  OutDataType=sfix(16)  OutScaling=2^0
  Data Store Memory12 : DataStoreMemory  DataStoreName=a2  InitialValue=Elements{id}.a2  OutDataType=sfix(16)  OutScaling=2^0
  Data Store Memory13 : DataStoreMemory  DataStoreName=ek11  InitialValue=Elements{id}.ek11  OutDataType=sfix(16)  OutScaling=2^0
  Data Store Memory14 : DataStoreMemory  DataStoreName=eal  InitialValue=Elements{id}.eal  OutDataType=sfix(16)  OutScaling=2^0
  Data Store Memory15 : DataStoreMemory  DataStoreName=ek12  InitialValue=Elements{id}.ek12  OutDataType=sfix(16)  OutScaling=2^0
  Data Store Memory16 : DataStoreMemory  DataStoreName=ek22h  InitialValue=Elements{id}.ek22h  OutDataType=sfix(16)  OutScaling=2^0
  Data Store Memory17 : DataStoreMemory  DataStoreName=ek22  InitialValue=Elements{id}.ek22  OutDataType=sfix(16)  OutScaling=2^0
  Data Store Memory18 : DataStoreMemory  DataStoreName=pmx  InitialValue=Elements{id}.pmx  OutDataType=sfix(16)  OutScaling=2^0
  Data Store Memory19 : DataStoreMemory  DataStoreName=fl  InitialValue=Elements{id}.fl  OutDataType=sfix(16)  OutScaling=2^0
  Data Store Memory2 : DataStoreMemory  DataStoreName=Node2UX  InitialValue=Elements{id}.Nodes(2).UX  OutDataType=sfix(16)  OutScaling=2^0
  Data Store Memory20 : DataStoreMemory  DataStoreName=ek11h  InitialValue=Elements{id}.ek11h  OutDataType=sfix(16)  OutScaling=2^0
  Data Store Memory21 : DataStoreMemory  DataStoreName=pr21  InitialValue=Elements{id}.pr21  OutDataType=sfix(16)  OutScaling=2^0
  Data Store Memory22 : DataStoreMemory  DataStoreName=pr12  InitialValue=Elements{id}.pr12  OutDataType=sfix(16)  OutScaling=2^0
  Data Store Memory23 : DataStoreMemory  DataStoreName=sina  InitialValue=Elements{id}.sina  OutDataType=sfix(16)  OutScaling=2^0
  Data Store Memory24 : DataStoreMemory  DataStoreName=psh  InitialValue=Elements{id}.psh  OutDataType=sfix(16)  OutScaling=2^0
  Data Store Memory25 : DataStoreMemory  DataStoreName=bmy  InitialValue=Elements{id}.bmy  OutDataType=sfix(16)  OutScaling=2^0
  Data Store Memory3 : DataStoreMemory  DataStoreName=Node1THETA  InitialValue=Elements{id}.Nodes(1).THETA  OutDataType=sfix(16)  OutScaling=2^0
  Data Store Memory4 : DataStoreMemory  DataStoreName=Node2UY  InitialValue=Elements{id}.Nodes(2).UY  OutDataType=sfix(16)  OutScaling=2^0
  Data Store Memory6 : DataStoreMemory  DataStoreName=Node1UX  InitialValue=Elements{id}.Nodes(1).UX  OutDataType=sfix(16)  OutScaling=2^0
  Data Store Memory7 : DataStoreMemory  DataStoreName=Node1UY  InitialValue=Elements{id}.Nodes(1).UY  OutDataType=sfix(16)  OutScaling=2^0
  Data Store Memory8 : DataStoreMemory  DataStoreName=Node2THETA  InitialValue=Elements{id}.Nodes(2).THETA  OutDataType=sfix(16)  OutScaling=2^0
  Data Store Memory9 : DataStoreMemory  DataStoreName=ksurf  InitialValue=Elements{id}.ksurf  OutDataType=sfix(16)  OutScaling=2^0
  Data Store Read1 : DataStoreRead  DataStoreName=Node1UX  SampleTime=-1
  Data Store Read13 : DataStoreRead  DataStoreName=Node2UY  SampleTime=-1
  Data Store Read15 : DataStoreRead  DataStoreName=a1  SampleTime=-1
  Data Store Read16 : DataStoreRead  DataStoreName=a2  SampleTime=-1
  Data Store Read17 : DataStoreRead  DataStoreName=cosa  SampleTime=-1
  Data Store Read18 : DataStoreRead  DataStoreName=eal  SampleTime=-1
  Data Store Read19 : DataStoreRead  DataStoreName=ek11  SampleTime=-1
  Data Store Read2 : DataStoreRead  DataStoreName=Node2THETA  SampleTime=-1
  Data Store Read20 : DataStoreRead  DataStoreName=ksurf  SampleTime=-1
  Data Store Read21 : DataStoreRead  DataStoreName=ek11h  SampleTime=-1
  Data Store Read22 : DataStoreRead  DataStoreName=ek12  SampleTime=-1
  Data Store Read23 : DataStoreRead  DataStoreName=ek22  SampleTime=-1
  Data Store Read24 : DataStoreRead  DataStoreName=ek22h  SampleTime=-1
  Data Store Read25 : DataStoreRead  DataStoreName=fl  SampleTime=-1
  Data Store Read26 : DataStoreRead  DataStoreName=pmx  SampleTime=-1
  Data Store Read27 : DataStoreRead  DataStoreName=pr12  SampleTime=-1
  Data Store Read28 : DataStoreRead  DataStoreName=pr21  SampleTime=-1
  Data Store Read29 : DataStoreRead  DataStoreName=psh  SampleTime=-1
  Data Store Read30 : DataStoreRead  DataStoreName=sina  SampleTime=-1
  Data Store Read31 : DataStoreRead  DataStoreName=bmy  SampleTime=-1
  Data Store Read4 : DataStoreRead  DataStoreName=Node1UY  SampleTime=-1
  Data Store Read8 : DataStoreRead  DataStoreName=Node1THETA  SampleTime=-1
  Data Store Read9 : DataStoreRead  DataStoreName=Node2UX  SampleTime=-1
  Element : Outport  OutDataType=sfix(16)  OutScaling=2^0
  a1 : Outport  Port=2  OutDataType=sfix(16)  OutScaling=2^0
  a2 : Outport  Port=3  OutDataType=sfix(16)  OutScaling=2^0
  pmx : Outport  Port=4  OutDataType=sfix(16)  OutScaling=2^0
  bmy : Outport  Port=5  OutDataType=sfix(16)  OutScaling=2^0
  wires:
  Data Store Read2/1 -> Bus Creator/19
  Data Store Read13/1 -> Bus Creator/18
  Data Store Read9/1 -> Bus Creator/17
  Data Store Read8/1 -> Bus Creator/16
  Data Store Read4/1 -> Bus Creator/15
  Data Store Read1/1 -> Bus Creator/14
  Bus Creator/1 -> Element/1
  Data Store Read20/1 -> Bus Creator/1  "ksurf"
  Data Store Read17/1 -> Bus Creator/2  "cosa"
  Data Store Read18/1 -> Bus Creator/3  "eal"
  Data Store Read19/1 -> Bus Creator/4  "ek11"
  Data Store Read21/1 -> Bus Creator/5  "ek11h"
  Data Store Read22/1 -> Bus Creator/6  "ek12"
  Data Store Read23/1 -> Bus Creator/7  "ek22"
  Data Store Read24/1 -> Bus Creator/8  "ek22h"
  Data Store Read25/1 -> Bus Creator/9  "fl"
  Data Store Read27/1 -> Bus Creator/10  "pr12"
  Data Store Read28/1 -> Bus Creator/11  "pr21"
  Data Store Read29/1 -> Bus Creator/12  "psh"
  Data Store Read30/1 -> Bus Creator/13  "sina"
  Data Store Read15/1 -> a1/1  "a1"
  Data Store Read16/1 -> a2/1  "a2"
  Data Store Read26/1 -> pmx/1  "pmx"
  Data Store Read31/1 -> bmy/1  "bmy"
